simulink model "model"  (R2020b)
settings: Solver=ode4  StartTime=0.0  StopTime=100  FixedStep=time_step  RelTol=1e-3
values from neighbouring files (symbols this model uses):
  A = [-831.638321287  -19.9481863665  0; 38.8007791523  -0.119086845313  0; 0  1  0]    [example_measurements.mat]    (also in example_params.m = [0 1)
  B = [5583.68566748 0 0]    [example_measurements.mat]    (also in example_params.m = [0)
  C = [0 0 1]    [example_measurements.mat]    (also in example_params.m = [2 0])
  G1 = G1_vec    [getG1G2.m]
  G2 = G2_vec    [getG1G2.m]
  input_noise_power = 0.000    (= 0)    [example_model_observation.m]
  n = s(1)    [calculateJ.m]    (also in example_calculate_Js.m = length(A); example_model_observation.m = length(A); example_real_data.m = length(A); example_use.m = length(A))
  output_noise_power = 0.000    (= 0)    [example_model_observation.m]
  time_samples = 0:0.01:T    [example_calculate_Js.m]    (also in example_model_observation.m = 0:time_step:T; example_real_data.m = 0:time_step:T; example_use.m = 0:0.01:0.5; getoptiG1G2.m = 0:time_step:T)
  time_samples_count = length(time_samples)    [example_model_observation.m]    (also in example_real_data.m)
  time_step = 0.01    [example_model_observation.m]    (also in example_real_data.m = time(2) - time(1))
  x0 = ones(1, n)    [example_model_observation.m]    (also in example_real_data.m = zeros(1, n))
libraries: simulink x4
settings Model: Creator=Ja  LastModifiedBy=Mario
settings DebuggingCC: UnconnectedInputMsg=none  UnconnectedOutputMsg=none  UnconnectedLineMsg=none  SFMachineParentedDataDiag=error
settings ModelReferenceCC: EnableRefExpFcnMdlSchedulingChecks=off

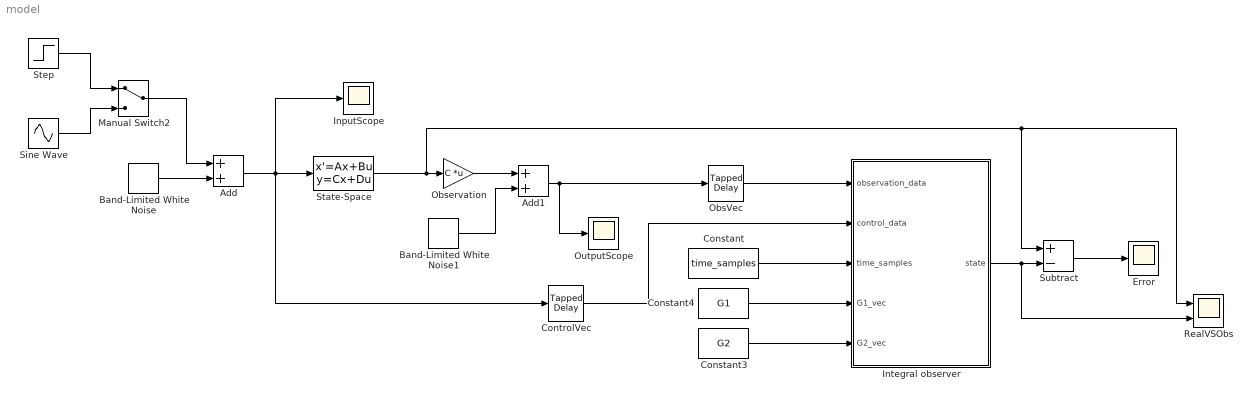
== system model ==
  Add : Sum
  Add1 : Sum
  Band-Limited White Noise : simulink/Sources/Band-Limited White Noise  Cov=[input_noise_power]  Ts=time_step  seed=[23341]
  Band-Limited White Noise1 : simulink/Sources/Band-Limited White Noise  Cov=[output_noise_power]  Ts=time_step  seed=[23341]
  Constant : Constant  Value=time_samples
  Constant3 : Constant  Value=G2
  Constant4 : Constant  Value=G1
  ControlVec : simulink/Discrete/Tapped Delay  vinit=0.0  samptime=-1  NumDelays=time_samples_count  DelayOrder=Oldest  includeCurrent=off
  Error : Scope
  InputScope : Scope
  Integral observer : MATLAB Function  TreatAsAtomicUnit=on
  Manual Switch2 : ManualSwitch
  ObsVec : simulink/Discrete/Tapped Delay  vinit=0.0  samptime=-1  NumDelays=time_samples_count  DelayOrder=Oldest  includeCurrent=off
  Observation : Gain  Gain=C  Multiplication=Matrix(K*u)
  OutputScope : Scope
  RealVSObs : Scope  NumInputPorts=2
  Sine Wave : Sin  SampleTime=0
  State-Space : StateSpace  A=A  B=B  C=eye(n)  D=zeros(n, inputsize)  InitialCondition=x0
  Step : Step  Time=3  SampleTime=0
  Subtract : Sum  Inputs=+-
  wires:
  Add1/1 -> ObsVec/1, OutputScope/1
  Constant3/1 -> Integral observer/5(G2_vec)
  ControlVec/1 -> Integral observer/2(control_data)
  State-Space/1 -> RealVSObs/1, Subtract/1, Observation/1
  Integral observer/1(state) -> RealVSObs/2, Subtract/2
  ObsVec/1 -> Integral observer/1(observation_data)
  Constant/1 -> Integral observer/3(time_samples)
  Constant4/1 -> Integral observer/4(G1_vec)
  Band-Limited White Noise/1 -> Add/2
  Band-Limited White Noise1/1 -> Add1/2
  Observation/1 -> Add1/1
  Step/1 -> Manual Switch2/1
  Sine Wave/1 -> Manual Switch2/2
  Manual Switch2/1 -> Add/1
  Subtract/1 -> Error/1
  Add/1 -> ControlVec/1, InputScope/1, State-Space/1

== matlab function model/Integral observer ==
  data: observation_data input; state output size=n; control_data input; time_samples input; G1_vec input; G2_vec input
function state = fcn(observation_data, control_data, time_samples,G1_vec, G2_vec)
    % funkcja licząca numerycznie obserwacje
    
    G1xY = squeeze(bsxfun(@times,G1_vec,reshape(observation_data, 1, 1, [])));
    G2xU = squeeze(bsxfun(@times,G2_vec,reshape(control_data, 1, 1, [])));
    
    state_obs = trapz(time_samples, G1xY, 2);
    control_obs = trapz(time_samples, G2xU, 2);
    
    state = state_obs + control_obs;
end
